simulink model "LineDetection"  (Simulink 6.5)
settings: Solver=ode45  StartTime=0.0  StopTime=0  RelTol=1e-3
undefined symbols (not defined in the file or in its folder): jet
libraries: viptransforms x2, dspindex x2, vipsrcs x1, vipanalysis x1, vipstatistics x1, viptextngfix x1, vipsnks x1
settings Model: Creator=greith  LastModifiedBy=jacobf

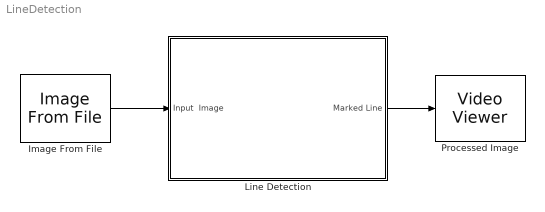
== system LineDetection ==
  Image From File : vipsrcs/Image From File  DialogController=vipDDGCreate  DialogControllerArgs=DataTag0  SystemSampleTime=-1  FileName=D:\4Graham\Image Processing\Lane Detection\SIM\circuit.tif  Ts=1  ImageDataType=Inherit from input image  Signed=on  WordLength=16  sdImageDataType=uint(8)  FractionLengthMode=User-defined  FractionLength=15  OutPortLabels=R|G|B
  Line Detection : Subsystem
  Processed Image : vipsnks/Video Viewer  inputType=Intensity  useColorMap=off  colormapValue=jet(256);  specRange=off  minInputVal=0  maxInputVal=255  FigPos=[622 594 676 470]  AxisZoom=on  trueSizedOnce=on
  wires:
  Line Detection/1(Marked Line) -> Processed Image/1
  Image From File/1 -> Line Detection/1(Input  Image)

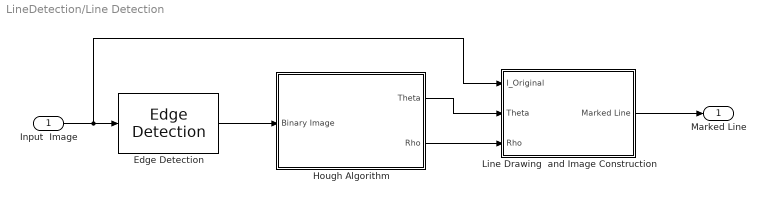
== system LineDetection/Line Detection ==
  Input  Image : Inport
  Edge Detection : vipanalysis/Edge Detection  DialogController=vipDDGCreate  DialogControllerArgs=DataTag1  method=Sobel  outputType=Binary image  userDefinedThreshold=on  thresholdSource=Specify via dialog  threshold=20  thresholdTuning=2  edgeThinning=off  threshold_canny=[0.25 0.60]  autoPercent=70  sigma=1  prodOutputMode=Binary point scaling  prodOutputWordLength=32  prodOutputFracLength=8  roundingMode=Floor  overflowMode=off
  Hough Algorithm : Subsystem
  Line Drawing  and Image Construction : Subsystem
  Marked Line : Outport
  wires:
  Edge Detection/1 -> Hough Algorithm/1(Binary Image)
  Hough Algorithm/2(Rho) -> Line Drawing  and Image Construction/3(Rho)
  Line Drawing  and Image Construction/1(Marked Line) -> Marked Line/1
  Hough Algorithm/1(Theta) -> Line Drawing  and Image Construction/2(Theta)
  Input  Image/1 -> Edge Detection/1, Line Drawing  and Image Construction/1(I_Original)

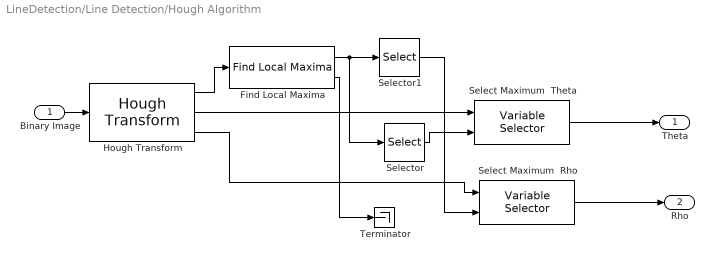
== system LineDetection/Line Detection/Hough Algorithm ==
  Binary Image : Inport
  Find Local Maxima : vipstatistics/Find Local Maxima  num_peaks=1  nhood_size=[5 7]  src_thresh=Specify via dialog  threshold=10  inputIsHough=on  dt_peak=uint32  dt_count=uint32
  Hough Transform : viptransforms/Hough Transform  DialogController=vipDDGCreate  DialogControllerArgs=DataTag2  theta_res=pi/360  rho_res=1  out_theta_rho=on  outdtmode=double  firstCoeffMode=Binary point scaling  firstCoeffWordLength=16  firstCoeffFracLength=14  secondCoeffMode=Binary point scaling  secondCoeffWordLength=32  secondCoeffFracLength=16  outputMode=Binary point scaling  outputWordLength=16  outputFracLength=0  accumMode=Binary point scaling  accumWordLength=32  accumFracLength=20  prodOutputMode=Binary point scaling  prodOutputWordLength=32  prodOutputFracLength=20  memoryMode=Binary point scaling  memoryWordLength=32  memoryFracLength=16  roundingMode=Nearest  overflowMode=on
  Select Maximum  Rho : dspindex/Variable Selector  NumInputs=1  rowsOrCols=Columns  IdxMode=Variable  Elements=[1 3]  ZerOneIdxMode=Zero-based  errmode=Clip Index  FillMode=on  FillValues=0
  Select Maximum  Theta : dspindex/Variable Selector  NumInputs=1  rowsOrCols=Columns  IdxMode=Variable  Elements=[1 3]  ZerOneIdxMode=Zero-based  errmode=Clip Index  FillMode=on  FillValues=0
  Selector : Selector  InputType=Vector  IndexMode=Zero-based  ElementSrc=Internal  Elements=1  RowSrc=Internal  Rows=1  ColumnSrc=Internal  Columns=1  InputPortWidth=2  IndexIsStartValue=off
  Selector1 : Selector  InputType=Vector  IndexMode=Zero-based  ElementSrc=Internal  Elements=0  RowSrc=Internal  Rows=1  ColumnSrc=Internal  Columns=1  InputPortWidth=2  IndexIsStartValue=off
  Terminator : Terminator
  Theta : Outport
  Rho : Outport  Port=2
  wires:
  Find Local Maxima/1 -> Selector1/1, Selector/1
  Find Local Maxima/2 -> Terminator/1
  Selector1/1 -> Select Maximum  Rho/2
  Selector/1 -> Select Maximum  Theta/2
  Hough Transform/3 -> Select Maximum  Rho/1
  Hough Transform/1 -> Find Local Maxima/1
  Hough Transform/2 -> Select Maximum  Theta/1
  Binary Image/1 -> Hough Transform/1
  Select Maximum  Theta/1 -> Theta/1
  Select Maximum  Rho/1 -> Rho/1

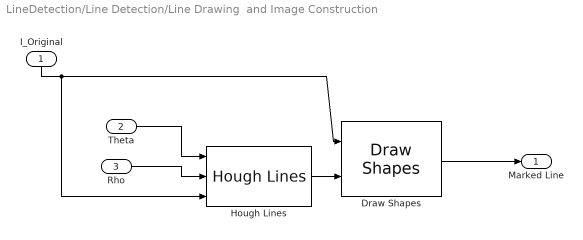
== system LineDetection/Line Detection/Line Drawing  and Image Construction ==
  I_Original : Inport  Orientation=down
  Theta : Inport  Port=2
  Rho : Inport  Port=3
  Draw Shapes : viptextngfix/Draw Shapes  DialogController=vipDDGCreate  DialogControllerArgs=DataTag3  inType=Intensity  shape=Lines  fill=off  display=White  intensity=200  color=[200 255 100]  opacity=0.6  viewport=Entire image  antialiasing=off
  Hough Lines : viptransforms/Hough Lines  DialogController=vipDDGCreate  DialogControllerArgs=DataTag4  sineCompMethod=Trigonometric function  thetaRes=pi/180  firstCoeffMode=Specify word length  firstCoeffWordLength=16  firstCoeffFracLength=15  prodOutputMode=Binary point scaling  prodOutputWordLength=32  prodOutputFracLength=16  roundingMode=Nearest  overflowMode=on
  Marked Line : Outport
  wires:
  Hough Lines/1 -> Draw Shapes/2
  I_Original/1 -> Draw Shapes/1, Hough Lines/3
  Theta/1 -> Hough Lines/1
  Draw Shapes/1 -> Marked Line/1
  Rho/1 -> Hough Lines/2
